simulink model "PTEngineCU"  (Simulink 10.3)
settings: Solver=ode45  StartTime=0.0  StopTime=inf  RelTol=1e-3  EnableMultiTasking=on
PreLoadFcn:
  | Trq_x = [500.0, 600.0, 700.0, 800.0, 1000.0, 2000.0, 3000.0, 4000.0, 4500.0, 5000.0, 6000.0, 7000.0, 8000.0];
  | TrqFull_y = [10.0, 40.0, 70.0, 95.0, 120.0, 145.0, 165.0, 180.0, 185.0, 182.0, 168.0, 130.0, 0.0];
  | 
  | TrqDrag_y = [-10.0, -10.0, -10.0, -10.0, -10.0, -20.0, -30.0, -40.0, -45.0, -50.0, -60.0, -70.0, -80.0];
  | 
  | TrqOpt_y = [0.0, 0.0, 0.0, 0.0, 0.0, 0.0, 0.0, 0.0, 0.0, 0.0, 0.0, 0.0, 0.0];
InitFcn:
  | Trq_x = [500.0, 600.0, 700.0, 800.0, 1000.0, 2000.0, 3000.0, 4000.0, 4500.0, 5000.0, 6000.0, 7000.0, 8000.0];
  | TrqFull_y = [10.0, 40.0, 70.0, 95.0, 120.0, 145.0, 165.0, 180.0, 185.0, 182.0, 168.0, 130.0, 0.0];
  | 
  | TrqDrag_y = [-10.0, -10.0, -10.0, -10.0, -10.0, -20.0, -30.0, -40.0, -45.0, -50.0, -60.0, -70.0, -80.0];
  | 
  | TrqOpt_y = [0.0, 0.0, 0.0, 0.0, 0.0, 0.0, 0.0, 0.0, 0.0, 0.0, 0.0, 0.0, 0.0];
libraries: simulink x7, CarMaker4SL x4
(part 3 of 3)

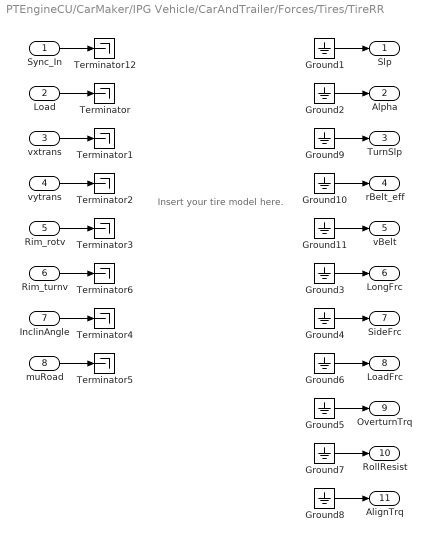
== system PTEngineCU/CarMaker/IPG Vehicle/CarAndTrailer/Forces/Tires/TireRR ==
  note: Insert your tire model here.
  Sync_In : Inport
  Load : Inport  Port=2
  vxtrans : Inport  Port=3
  vytrans : Inport  Port=4
  Rim_rotv : Inport  Port=5
  Rim_turnv : Inport  Port=6
  InclinAngle : Inport  Port=7
  muRoad : Inport  Port=8
  Ground{1..11} (11 alike) : Ground
  Terminator{,1..6,12} (8 alike) : Terminator
  Slp : Outport  VectorParamsAs1DForOutWhenUnconnected=off
  Alpha : Outport  Port=2  VectorParamsAs1DForOutWhenUnconnected=off
  TurnSlp : Outport  Port=3  VectorParamsAs1DForOutWhenUnconnected=off
  rBelt_eff : Outport  Port=4  VectorParamsAs1DForOutWhenUnconnected=off
  vBelt : Outport  Port=5  VectorParamsAs1DForOutWhenUnconnected=off
  LongFrc : Outport  Port=6  VectorParamsAs1DForOutWhenUnconnected=off
  SideFrc : Outport  Port=7  VectorParamsAs1DForOutWhenUnconnected=off
  LoadFrc : Outport  Port=8  VectorParamsAs1DForOutWhenUnconnected=off
  OverturnTrq : Outport  Port=9  VectorParamsAs1DForOutWhenUnconnected=off
  RollResist : Outport  Port=10  VectorParamsAs1DForOutWhenUnconnected=off
  AlignTrq : Outport  Port=11  VectorParamsAs1DForOutWhenUnconnected=off
  wires:
  Ground11/1 -> vBelt/1
  Ground10/1 -> rBelt_eff/1
  Ground9/1 -> TurnSlp/1
  Rim_turnv/1 -> Terminator6/1
  Sync_In/1 -> Terminator12/1
  Ground2/1 -> Alpha/1
  Ground3/1 -> LongFrc/1
  Ground4/1 -> SideFrc/1
  Ground5/1 -> OverturnTrq/1
  vxtrans/1 -> Terminator1/1
  vytrans/1 -> Terminator2/1
  Rim_rotv/1 -> Terminator3/1
  InclinAngle/1 -> Terminator4/1
  muRoad/1 -> Terminator5/1
  Load/1 -> Terminator/1
  Ground1/1 -> Slp/1
  Ground6/1 -> LoadFrc/1
  Ground7/1 -> RollResist/1
  Ground8/1 -> AlignTrq/1

== system PTEngineCU/CarMaker/IPG Vehicle/PowerTrain/ECU Example/MyEngineCU/Enabled Subsystem1 ==
  rotv_off : Inport
  Engine_on last cycle : Inport  Port=2
  rotv_idle : Inport  Port=3
  rotv : Inport  Port=4
  Enable : EnablePort
  Engine off : Subsystem  TreatAsAtomicUnit=on
  Engine on : Subsystem  TreatAsAtomicUnit=on
  Engine on? : If  NumInputs=3  IfExpression=u1 > u2  ElseIfExpressions=u1 < u3
  If Action Subsystem2 : Subsystem  TreatAsAtomicUnit=on
  Merge : Merge  Inputs=3
  Engine_on : Outport  VectorParamsAs1DForOutWhenUnconnected=off
  wires:
  Engine off/1(Engine_off) -> Merge/2
  Engine on/1(Engine_on) -> Merge/1
  If Action Subsystem2/1(Engine_on) -> Merge/3
  Merge/1 -> Engine_on/1
  Engine_on last cycle/1 -> If Action Subsystem2/1(Engine_on last cycle)
  Engine on?/3 -> If Action Subsystem2/Action
  Engine on?/2 -> Engine off/Action
  Engine on?/1 -> Engine on/Action
  rotv_off/1 -> Engine on?/3
  rotv_idle/1 -> Engine on?/2
  rotv/1 -> Engine on?/1

== system PTEngineCU/CarMaker/IPG Vehicle/PowerTrain/ECU Example/MyEngineCU/Return Zero ==
  Enable : EnablePort
  Bus Creator : BusCreator  Inputs=6
  Constant : Constant  Value=0
  Constant1 : Constant  Value=0
  Constant{2..5} (4 alike) : Constant  Value=0.0
  Outputs Retrun Zero : Outport  SampleTime=0.001  InitialOutput=0  VectorParamsAs1DForOutWhenUnconnected=off
  wires:
  Constant5/1 -> Bus Creator/6  "TrqOpt"
  Constant4/1 -> Bus Creator/5  "TrqDrag"
  Constant3/1 -> Bus Creator/4  "TrqFull"
  Constant2/1 -> Bus Creator/3  "Load"
  Constant1/1 -> Bus Creator/2  "FuelCutOff"
  Constant/1 -> Bus Creator/1  "Engine_on"
  Bus Creator/1 -> Outputs Retrun Zero/1

== system PTEngineCU/CarMaker/IPG Vehicle/PowerTrain/ECU Example/MyEngineCU/Return Zero1 ==
  Enable : EnablePort
  Bus Creator : BusCreator  Inputs=6
  Constant : Constant  Value=0
  Constant1 : Constant  Value=0
  Constant{2..5} (4 alike) : Constant  Value=0.0
  Outputs Retrun Zero : Outport  SampleTime=0.001  InitialOutput=0  VectorParamsAs1DForOutWhenUnconnected=off
  wires:
  Bus Creator/1 -> Outputs Retrun Zero/1
  Constant/1 -> Bus Creator/1  "Engine_on"
  Constant1/1 -> Bus Creator/2  "FuelCutOff"
  Constant2/1 -> Bus Creator/3  "Load"
  Constant3/1 -> Bus Creator/4  "TrqFull"
  Constant4/1 -> Bus Creator/5  "TrqDrag"
  Constant5/1 -> Bus Creator/6  "TrqOpt"

== system PTEngineCU/CarMaker/IPG Vehicle/PowerTrain/ECU Example/MyEngineCU/if Engine_on ==
  Engin_on : Inport
  Mappings : Inport  Port=2
  rotv_idle : Inport  Port=3
  rotv : Inport  Port=4
  Load : Inport  Port=5
  FuelCutOff : Inport  Port=6
  set_ISC : Inport  Port=7
  Enable : EnablePort
  == NOTSET : simulink/Logic and Bit Operations/Compare To Constant  relop===  const=-9999  OutDataTypeStr=uint8  ZeroCross=off
  Bus Creator : BusCreator  Inputs=6
  Bus Selector4 : BusSelector  OutputSignals=TrqFull,TrqDrag,TrqOpt
  Constant : Constant  Value=0.0
  FuelCutOff Function : Subsystem
  Gain : Gain
  Idle Speed Control : Subsystem
  Switch : Switch  Criteria=u2 ~= 0
  TrqFull & TrqDrag & TrqOpt : Subsystem
  Outputs : Outport  VectorParamsAs1DForOutWhenUnconnected=off
  wires:
  Gain/1 -> Bus Creator/1  "Engine_on"
  Bus Selector4/3 -> Bus Creator/6  "<TrqOpt>"
  Bus Selector4/2 -> Bus Creator/5  "<TrqDrag>"
  Bus Selector4/1 -> Bus Creator/4  "<TrqFull>"
  FuelCutOff Function/2(Load1) -> Bus Creator/3  "Load"
  FuelCutOff Function/1(FuelCutOff1) -> Bus Creator/2  "FuelCutOff"
  Engin_on/1 -> Gain/1
  Switch/1 -> Idle Speed Control/3(Load)  "Load"
  set_ISC/1 -> Idle Speed Control/2(set_ISC)
  rotv_idle/1 -> Idle Speed Control/1(rotv_idle)
  Idle Speed Control/1(Load_out) -> FuelCutOff Function/2(Load)
  FuelCutOff/1 -> FuelCutOff Function/1(FuelCutOff)
  TrqFull & TrqDrag & TrqOpt/1(Trg) -> Bus Selector4/1
  Constant/1 -> Switch/1
  == NOTSET/1 -> Switch/2
  Load/1 -> Switch/3, == NOTSET/1
  rotv/1 -> Idle Speed Control/4(rotv), FuelCutOff Function/3(rotv), TrqFull & TrqDrag & TrqOpt/1(rotv)
  Mappings/1 -> TrqFull & TrqDrag & TrqOpt/2(Mappings)
  Bus Creator/1 -> Outputs/1

== system PTEngineCU/CarMaker/IPG Vehicle/PowerTrain/ECU Example/PTEngineCU_In/CreateBus ECU_CfgIF ==
  In : Inport
  BusCreator : BusCreator  Inputs=4
  Demux : Demux
      settings: DisplayOption=none
  Out : Outport  VectorParamsAs1DForOutWhenUnconnected=off
  wires:
  Demux/4 -> BusCreator/4  "ECU_Cfg rotv_opt"
  Demux/3 -> BusCreator/3  "ECU_Cfg rotv_idle"
  Demux/2 -> BusCreator/2  "ECU_Cfg rotv_max"
  Demux/1 -> BusCreator/1  "ECU_Cfg rotv_off"
  BusCreator/1 -> Out/1
  In/1 -> Demux/1

== system PTEngineCU/CarMaker/IPG Vehicle/PowerTrain/ECU Example/PTEngineCU_In/CreateBus ECU_IF Input ==
  In : Inport
  BusCreator : BusCreator  Inputs=10
  Demux : Demux  Outputs=10
      settings: DisplayOption=none
  Out : Outport  VectorParamsAs1DForOutWhenUnconnected=off
  wires:
  Demux/10 -> BusCreator/10  "ECU FuelFlow"
  Demux/9 -> BusCreator/9  "ECU rot"
  Demux/8 -> BusCreator/8  "ECU rotv"
  Demux/7 -> BusCreator/7  "ECU rotv_trg"
  Demux/6 -> BusCreator/6  "ECU Trq"
  Demux/5 -> BusCreator/5  "ECU Trq_trg"
  Demux/4 -> BusCreator/4  "ECU Load"
  Demux/3 -> BusCreator/3  "ECU FuelCutOff"
  Demux/2 -> BusCreator/2  "ECU set_ISC"
  Demux/1 -> BusCreator/1  "ECU Ignition"
  BusCreator/1 -> Out/1
  In/1 -> Demux/1

== system PTEngineCU/CarMaker/IPG Vehicle/PowerTrain/ECU Example/MyEngineCU/Enabled Subsystem1/Engine off ==
  Action Port : ActionPort
  Constant : Constant  Value=0
  Engine_off : Outport  InitialOutput=0  VectorParamsAs1DForOutWhenUnconnected=off
  wires:
  Constant/1 -> Engine_off/1

== system PTEngineCU/CarMaker/IPG Vehicle/PowerTrain/ECU Example/MyEngineCU/Enabled Subsystem1/Engine on ==
  Action Port : ActionPort
  Constant : Constant
  Engine_on : Outport  InitialOutput=1  VectorParamsAs1DForOutWhenUnconnected=off
  wires:
  Constant/1 -> Engine_on/1

== system PTEngineCU/CarMaker/IPG Vehicle/PowerTrain/ECU Example/MyEngineCU/Enabled Subsystem1/If Action Subsystem2 ==
  Engine_on last cycle : Inport
  Action Port : ActionPort
  Engine_on : Outport  VectorParamsAs1DForOutWhenUnconnected=off
  wires:
  Engine_on last cycle/1 -> Engine_on/1

== system PTEngineCU/CarMaker/IPG Vehicle/PowerTrain/ECU Example/MyEngineCU/if Engine_on/FuelCutOff Function ==
  FuelCutOff : Inport
  Load : Inport  Port=2
  rotv : Inport  Port=3
  If : If  IfExpression=u1 == 1  ElseIfExpressions=u1 == -99999
  If Action Subsystem : Subsystem  TreatAsAtomicUnit=on
  If Action Subsystem1 : Subsystem  TreatAsAtomicUnit=on
  If Action Subsystem2 : Subsystem  TreatAsAtomicUnit=on
  Merge : Merge  Inputs=3
  Merge1 : Merge  Inputs=3
  Read CM Parameter : CarMaker4SL/Read CM Parameter  xfile=Vehicle  xkey=PowerTrain.ECU.FuelCutOff  xnout=1  xdefaults=1600  xmuxed=on  xstime=Continuous
  rpm2radsec : Gain  Gain=0.104719755
  FuelCutOff1 : Outport  VectorParamsAs1DForOutWhenUnconnected=off
  Load1 : Outport  Port=2  VectorParamsAs1DForOutWhenUnconnected=off
  wires:
  rpm2radsec/1 -> If Action Subsystem2/3(nFuelCutOff)
  Load/1 -> If Action Subsystem2/1(Load), If Action Subsystem1/2(Load)  "Load"
  FuelCutOff/1 -> If Action Subsystem1/1(FuelCutOff), If Action Subsystem/1(FuelCutOff), If/1
  Merge1/1 -> Load1/1
  Merge/1 -> FuelCutOff1/1
  Read CM Parameter/1 -> rpm2radsec/1
  rotv/1 -> If Action Subsystem2/2(rotv)
  If Action Subsystem/2(Load out) -> Merge1/1
  If Action Subsystem1/2(Load out) -> Merge1/2
  If Action Subsystem2/2(Load out) -> Merge1/3
  If Action Subsystem2/1(FuelCutOff out) -> Merge/3
  If Action Subsystem1/1(FuelCutOff out) -> Merge/2
  If Action Subsystem/1(FuelCutOff out) -> Merge/1
  If/1 -> If Action Subsystem/Action
  If/2 -> If Action Subsystem2/Action
  If/3 -> If Action Subsystem1/Action

== system PTEngineCU/CarMaker/IPG Vehicle/PowerTrain/ECU Example/MyEngineCU/if Engine_on/Idle Speed Control ==
  rotv_idle : Inport
  set_ISC : Inport  Port=2
  Load : Inport  Port=3
  rotv : Inport  Port=4
  Bus Creator1 : BusCreator  Inputs=2
  Bus Creator2 : BusCreator  Inputs=2
  Bus Selector : BusSelector  OutputSignals=Load_I,Load
  Constant2 : Constant  Value=0.0
  Load Copy : InportShadow  Port=3
  Load Copy2 : InportShadow  Port=3
  Memory1 : Memory  InheritSampleTime=on
  PI : Subsystem
  Saturation : Saturate  UpperLimit=1  LowerLimit=0
  Subtract : Sum  Inputs=+-
  Switch1 : Switch  Criteria=u2 ~= 0
  Switch2 : Switch  Criteria=u2 ~= 0
  if condition : Subsystem
  Load_out : Outport  VectorParamsAs1DForOutWhenUnconnected=off
  wires:
  Load Copy2/1 -> Switch1/3
  Load Copy/1 -> Bus Creator1/2
  PI/2(Load out) -> Bus Creator2/2
  Subtract/1 -> PI/3(drotv)  "drotv"
  Memory1/1 -> PI/1(ISCtrl.Load_I)
  Bus Selector/1 -> Memory1/1  "<Load_I>"
  Bus Selector/2 -> Switch1/1  "<Load>"
  PI/1(ISCtrl.Load_I out) -> Bus Creator2/1
  rotv/1 -> Subtract/2, if condition/2(rotv)
  rotv_idle/1 -> Subtract/1, if condition/1(rotv_idle)
  Saturation/1 -> Load_out/1
  Constant2/1 -> Bus Creator1/1  "Load_I"
  if condition/1(Boolean) -> Switch2/2
  Bus Creator2/1 -> Switch2/1
  Bus Creator1/1 -> Switch2/3
  Switch2/1 -> Bus Selector/1
  set_ISC/1 -> Switch1/2
  Load/1 -> PI/2(Load)
  Switch1/1 -> Saturation/1

== system PTEngineCU/CarMaker/IPG Vehicle/PowerTrain/ECU Example/MyEngineCU/if Engine_on/TrqFull & TrqDrag & TrqOpt ==
  rotv : Inport
  Mappings : Inport  Port=2
  Bus Creator1 : BusCreator  Inputs=3
  Bus Selector : BusSelector  OutputSignals=TrqFull,TrqDrag,TrqOpt
  Bus Selector1 : BusSelector  OutputSignals=x,z
  Bus Selector2 : BusSelector  OutputSignals=x,z
  Bus Selector3 : BusSelector  OutputSignals=x,z
  Lookup Table Dynamic : simulink/Lookup Tables/Lookup Table Dynamic  LookUpMeth=Interpolation-Use End Values  OutDataType=float('double')  OutScaling=2^-10  OutputDataTypeScalingMode=Specify via dialog  OutDataTypeStr=float('double')  DoSatur=off
  Lookup Table Dynamic1 : simulink/Lookup Tables/Lookup Table Dynamic  LookUpMeth=Interpolation-Use End Values  OutDataType=float('double')  OutScaling=2^-10  OutputDataTypeScalingMode=Specify via dialog  OutDataTypeStr=float('double')  DoSatur=off
  Lookup Table Dynamic2 : simulink/Lookup Tables/Lookup Table Dynamic  LookUpMeth=Interpolation-Use End Values  OutDataType=float('double')  OutScaling=2^-10  OutputDataTypeScalingMode=Specify via dialog  OutDataTypeStr=float('double')  DoSatur=off
  Trg : Outport  VectorParamsAs1DForOutWhenUnconnected=off
  wires:
  Mappings/1 -> Bus Selector/1
  Bus Creator1/1 -> Trg/1
  rotv/1 -> Lookup Table Dynamic2/1, Lookup Table Dynamic1/1, Lookup Table Dynamic/1
  Lookup Table Dynamic2/1 -> Bus Creator1/3  "TrqOpt"
  Lookup Table Dynamic1/1 -> Bus Creator1/2  "TrqDrag"
  Lookup Table Dynamic/1 -> Bus Creator1/1  "TrqFull"
  Bus Selector3/2 -> Lookup Table Dynamic2/3  "<z>"
  Bus Selector3/1 -> Lookup Table Dynamic2/2  "<x>"
  Bus Selector2/1 -> Lookup Table Dynamic1/2  "<x>"
  Bus Selector2/2 -> Lookup Table Dynamic1/3  "<z>"
  Bus Selector/3 -> Bus Selector3/1  "<TrqOpt>"
  Bus Selector/2 -> Bus Selector2/1  "<TrqDrag>"
  Bus Selector/1 -> Bus Selector1/1  "<TrqFull>"
  Bus Selector1/2 -> Lookup Table Dynamic/3  "<z>"
  Bus Selector1/1 -> Lookup Table Dynamic/2  "<x>"

== system PTEngineCU/CarMaker/IPG Vehicle/PowerTrain/ECU Example/MyEngineCU/if Engine_on/FuelCutOff Function/If Action Subsystem ==
  FuelCutOff : Inport
  Action Port : ActionPort
  Constant : Constant  Value=0.0
  FuelCutOff out : Outport  VectorParamsAs1DForOutWhenUnconnected=off
  Load out : Outport  Port=2  InitialOutput=0  VectorParamsAs1DForOutWhenUnconnected=off
  wires:
  FuelCutOff/1 -> FuelCutOff out/1
  Constant/1 -> Load out/1

== system PTEngineCU/CarMaker/IPG Vehicle/PowerTrain/ECU Example/MyEngineCU/if Engine_on/FuelCutOff Function/If Action Subsystem1 ==
  FuelCutOff : Inport
  Load : Inport  Port=2
  Action Port : ActionPort
  FuelCutOff out : Outport  VectorParamsAs1DForOutWhenUnconnected=off
  Load out : Outport  Port=2  VectorParamsAs1DForOutWhenUnconnected=off
  wires:
  FuelCutOff/1 -> FuelCutOff out/1
  Load/1 -> Load out/1

== system PTEngineCU/CarMaker/IPG Vehicle/PowerTrain/ECU Example/MyEngineCU/if Engine_on/FuelCutOff Function/If Action Subsystem2 ==
  Load : Inport
  rotv : Inport  Port=2
  nFuelCutOff : Inport  Port=3
  Action Port : ActionPort
  Compare To Constant : simulink/Logic and Bit Operations/Compare To Constant  relop=<=  const=1e-3  OutDataTypeStr=uint8  ZeroCross=off
  Constant : Constant
  Constant1 : Constant  Value=0
  Gain : Gain
  Logical Operator : Logic  AllPortsSameDT=off  OutDataTypeStr=boolean
  Relational Operator : RelationalOperator  OutDataTypeStr=boolean  RndMeth=Nearest
  Switch : Switch  Criteria=u2 ~= 0
  FuelCutOff out : Outport  VectorParamsAs1DForOutWhenUnconnected=off
  Load out : Outport  Port=2  VectorParamsAs1DForOutWhenUnconnected=off
  wires:
  Gain/1 -> Load out/1
  Constant1/1 -> Switch/3
  Constant/1 -> Switch/1
  Logical Operator/1 -> Switch/2
  Compare To Constant/1 -> Logical Operator/1
  Relational Operator/1 -> Logical Operator/2
  nFuelCutOff/1 -> Relational Operator/2
  rotv/1 -> Relational Operator/1
  Switch/1 -> FuelCutOff out/1
  Load/1 -> Gain/1, Compare To Constant/1

== system PTEngineCU/CarMaker/IPG Vehicle/PowerTrain/ECU Example/MyEngineCU/if Engine_on/Idle Speed Control/PI ==
  ISCtrl.Load_I : Inport
  Load : Inport  Port=2
  drotv : Inport  Port=3
  Add : Sum
  Add1 : Sum
  Constant : Constant  Value=0.0
  If : If  IfExpression=u1 < 1e-3
  If Action Subsystem : Subsystem  TreatAsAtomicUnit=on
  If Action Subsystem1 : Subsystem  TreatAsAtomicUnit=on
  Load1 : InportShadow  Port=2
  Max : MinMax  Function=max  Inputs=2
  Merge : Merge
  Merge1 : Merge
  Product : Product  RndMeth=Zero
  Read CM Parameter : CarMaker4SL/Read CM Parameter  xfile=Vehicle  xkey=PowerTrain.MyEngineCU.ISCtrl.P  xnout=1  xdefaults=0.1  xmuxed=on  xstime=Continuous
  Saturation : Saturate  UpperLimit=1  LowerLimit=0
  ISCtrl.Load_I out : Outport  VectorParamsAs1DForOutWhenUnconnected=off
  Load out : Outport  Port=2  VectorParamsAs1DForOutWhenUnconnected=off
  wires:
  Saturation/1 -> Add/2
  Load1/1 -> If/1
  Merge1/1 -> ISCtrl.Load_I out/1  "Load_I"
  If Action Subsystem1/1(ISCtrl.Load_I out) -> Merge1/1
  If Action Subsystem1/2(Load_I out) -> Merge/1
  If/1 -> If Action Subsystem1/Action
  If Action Subsystem/1(ISCtrl.Load_I out) -> Merge1/2
  If Action Subsystem/2(Load_I out) -> Merge/2
  Merge/1 -> Add1/1
  If/2 -> If Action Subsystem/Action
  ISCtrl.Load_I/1 -> If Action Subsystem1/1(ISCtrl.Load_I), If Action Subsystem/1(ISCtrl.Load_I)
  Load/1 -> Add/1
  Constant/1 -> Max/2
  Max/1 -> Add1/2
  Product/1 -> Max/1
  Read CM Parameter/1 -> Product/2
  drotv/1 -> If Action Subsystem1/2(drotv), If Action Subsystem/2(drotv), Product/1
  Add1/1 -> Saturation/1
  Add/1 -> Load out/1  "Load"

== system PTEngineCU/CarMaker/IPG Vehicle/PowerTrain/ECU Example/MyEngineCU/if Engine_on/Idle Speed Control/if condition ==
  rotv_idle : Inport
  rotv : Inport  Port=2
  Add : Sum
  Constant1 : Constant  Value=200.0
  Relational Operator : RelationalOperator  Operator=<  OutDataTypeStr=boolean  RndMeth=Nearest
  rpm2radsec : Gain  Gain=0.104719755
  Boolean : Outport  VectorParamsAs1DForOutWhenUnconnected=off
  wires:
  Add/1 -> Relational Operator/2
  rotv/1 -> Relational Operator/1
  Relational Operator/1 -> Boolean/1
  rotv_idle/1 -> Add/1
  Constant1/1 -> rpm2radsec/1
  rpm2radsec/1 -> Add/2

== system PTEngineCU/CarMaker/IPG Vehicle/PowerTrain/ECU Example/MyEngineCU/if Engine_on/Idle Speed Control/PI/If Action Subsystem ==
  ISCtrl.Load_I : Inport
  drotv : Inport  Port=2
  Action Port : ActionPort
  Add : Sum
  Constant : Constant
  Constant1 : Constant  Value=200.0
  Divide : Product  Inputs=*/
  Gain : Gain
  Product : Product  RndMeth=Zero
  Saturation : Saturate  UpperLimit=1  LowerLimit=0
  rpm2radsec : Gain  Gain=0.104719755
  ISCtrl.Load_I out : Outport  VectorParamsAs1DForOutWhenUnconnected=off
  Load_I out : Outport  Port=2  VectorParamsAs1DForOutWhenUnconnected=off
  wires:
  Gain/1 -> ISCtrl.Load_I out/1
  Saturation/1 -> Product/2
  Constant1/1 -> rpm2radsec/1
  rpm2radsec/1 -> Divide/2
  drotv/1 -> Divide/1
  Divide/1 -> Add/2
  Constant/1 -> Add/1
  Add/1 -> Saturation/1  "fac"
  Product/1 -> Load_I out/1
  ISCtrl.Load_I/1 -> Gain/1, Product/1

== system PTEngineCU/CarMaker/IPG Vehicle/PowerTrain/ECU Example/MyEngineCU/if Engine_on/Idle Speed Control/PI/If Action Subsystem1 ==
  ISCtrl.Load_I : Inport
  drotv : Inport  Port=2
  Action Port : ActionPort
  Add : Sum
  Gain : Gain
  Gain1 : Gain
  ISCtrl_I : Constant  Value=0.01
  Product : Product  RndMeth=Zero
  Saturation : Saturate  UpperLimit=1  LowerLimit=0
  ISCtrl.Load_I out : Outport  VectorParamsAs1DForOutWhenUnconnected=off
  Load_I out : Outport  Port=2  VectorParamsAs1DForOutWhenUnconnected=off
  wires:
  Gain1/1 -> Load_I out/1
  Gain/1 -> ISCtrl.Load_I out/1
  ISCtrl_I/1 -> Product/2
  drotv/1 -> Product/1
  Product/1 -> Add/1
  ISCtrl.Load_I/1 -> Add/2
  Saturation/1 -> Gain1/1, Gain/1
  Add/1 -> Saturation/1
